simulink model "schiefeebenehaftung"  (R2016a)
settings: Solver=VariableStepAuto  StartTime=0.0  StopTime=20  MaxStep=0.01  RelTol=1e-3
values from neighbouring files (symbols this model uses):
  g = 9.81    [schiefeebenehaftungskript.m]
  m = 20    [schiefeebenehaftungskript.m]
  mu = 0.4    [schiefeebenehaftungskript.m]
  mu0 = 0.6    [schiefeebenehaftungskript.m]
libraries: simulink x1
settings Model: Creator=NachtHemd  LastModifiedBy=NachtHemd

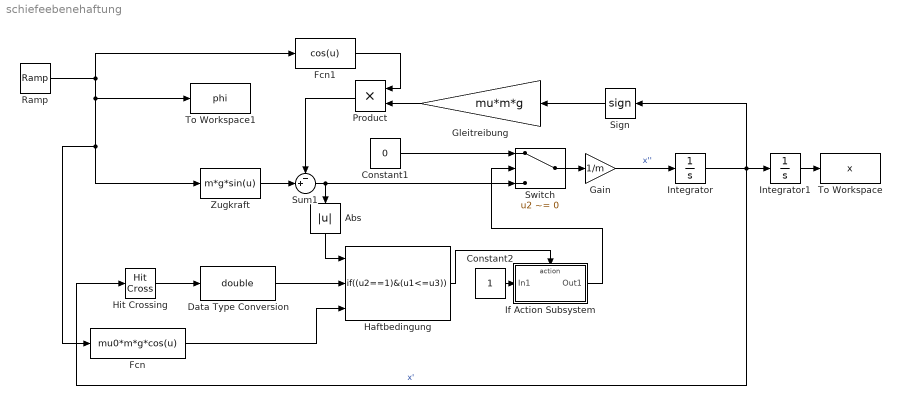
== system schiefeebenehaftung ==
  Abs : Abs  ZeroCross=off
  Constant1 : Constant  Value=0
  Constant2 : Constant
  Data Type Conversion : DataTypeConversion  OutDataTypeStr=double
  Fcn : Fcn  Expr=mu0*m*g*cos(u)
  Fcn1 : Fcn  Expr=cos(u)
  Gain : Gain  Gain=1/m
  Gleitreibung : Gain  Gain=mu*m*g
  Haftbedingung : If  NumInputs=3  IfExpression=(u2==1)&(u1<=u3)  ShowElse=off
  Hit Crossing : HitCross  ZeroCross=off
  If Action Subsystem : Subsystem  TreatAsAtomicUnit=on
  Integrator : Integrator
  Integrator1 : Integrator
  Product : Product
  Ramp : simulink/Sources/Ramp  slope=0.1  start=1  X0=0
  Sign : Signum  ZeroCross=off
  Sum1 : Sum  Inputs=-+|
  Switch : Switch  Criteria=u2 ~= 0
  To Workspace : ToWorkspace  VariableName=x  SaveFormat=Structure With Time  SampleTime=-1
  To Workspace1 : ToWorkspace  VariableName=phi  SaveFormat=Structure With Time  SampleTime=-1
  Zugkraft : Fcn  Expr=m*g*sin(u)
  wires:
  Gain/1 -> Integrator/1  "x''"
  Integrator/1 -> Hit Crossing/1, Sign/1, Integrator1/1  "x'"
  Switch/1 -> Gain/1
  Constant1/1 -> Switch/1
  Sign/1 -> Gleitreibung/1
  Sum1/1 -> Abs/1, Switch/3
  Fcn/1 -> Haftbedingung/3
  Haftbedingung/1 -> If Action Subsystem/Action
  Hit Crossing/1 -> Data Type Conversion/1
  Abs/1 -> Haftbedingung/1
  Data Type Conversion/1 -> Haftbedingung/2
  Constant2/1 -> If Action Subsystem/1(In1)
  If Action Subsystem/1(Out1) -> Switch/2
  Zugkraft/1 -> Sum1/2
  Integrator1/1 -> To Workspace/1
  Product/1 -> Sum1/1
  Gleitreibung/1 -> Product/2
  Ramp/1 -> To Workspace1/1, Fcn/1, Zugkraft/1, Fcn1/1
  Fcn1/1 -> Product/1

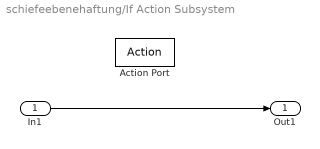
== system schiefeebenehaftung/If Action Subsystem ==
  In1 : Inport
  Action Port : ActionPort  InitializeStates=reset  ActionType=then
  Out1 : Outport  OutputWhenDisabled=reset  InitialOutput=0
  wires:
  In1/1 -> Out1/1
